simulink model "sudoku_PP_CEX2"  (R2017b)
settings: Solver=FixedStepDiscrete  StartTime=0.0  StopTime=10.0  FixedStep=0.200000  RelTol=1e-3
model workspace (MAT data in the model file):
  MCOS : class17 (value not decoded)
  already_pp = 1
  compositionalMap : struct (value not decoded)
  MCOS : class17 (value not decoded)
  MCOS : class17 (value not decoded)
  verificationResults : struct (value not decoded)
undefined symbols (not defined in the file): contractAfterSimulation, ContractAssumeBlock, contractBeforeSimulation, ContractBlock, ContractGuaranteeBlock, ContractValidatorBlock, saveValidatorParameters
(part 7 of 17)

== system sudoku_PP_CEX2/contract/guarantee/RowsValid/ForEach_newline_Subsystem/ForEach3/Vectorisvalid ==
  In1 : Inport
  Compare To Constant : Subsystem  AncestorBlock=|  TreatAsAtomicUnit=on  mask(Compare To Constant){relop===, const=1, OutDataTypeStr=boolean, ZeroCross=on}
      | simulink/Logic and Bit
      | Operations/Compare
      | To Constant
      mask prompts: relop "Simulink:masks:Operator_MP"; const "Simulink:masks:ConstantValue_MP"; OutDataTypeStr "Simulink:masks:OutputDataType_MP"; ZeroCross "Simulink:masks:EnableZerocrossingDetection_MP"
      mask help: Simulink:masks:CompareToConstant_MD
      mask init: same as sudoku_PP_CEX2/contract/guarantee/ColsValid/ForEach_newline_Subsystem/ForEach1/Vectorisvalid/Compare To Constant
      mask TypeOptions relop: == | ~= | < | <= | >= | >
      mask TypeOptions OutDataTypeStr: Simulink:masks:uint8 | Simulink:masks:boolean
      mask Callback ZeroCross: sl('zeroCrossEnable', gcbh);
      mask Display: disp(str)
  Compare To Constant1 : Subsystem  AncestorBlock=|  TreatAsAtomicUnit=on  mask(Compare To Constant){relop===, const=1, OutDataTypeStr=boolean, ZeroCross=on}
      | simulink/Logic and Bit
      | Operations/Compare
      | To Constant
      mask prompts: relop "Simulink:masks:Operator_MP"; const "Simulink:masks:ConstantValue_MP"; OutDataTypeStr "Simulink:masks:OutputDataType_MP"; ZeroCross "Simulink:masks:EnableZerocrossingDetection_MP"
      mask help: Simulink:masks:CompareToConstant_MD
      mask init: same as sudoku_PP_CEX2/contract/guarantee/ColsValid/ForEach_newline_Subsystem/ForEach1/Vectorisvalid/Compare To Constant
      mask TypeOptions relop: == | ~= | < | <= | >= | >
      mask TypeOptions OutDataTypeStr: Simulink:masks:uint8 | Simulink:masks:boolean
      mask Callback ZeroCross: sl('zeroCrossEnable', gcbh);
      mask Display: disp(str)
  Compare To Constant2 : Subsystem  AncestorBlock=|  TreatAsAtomicUnit=on  mask(Compare To Constant){relop===, const=1, OutDataTypeStr=boolean, ZeroCross=on}
      | simulink/Logic and Bit
      | Operations/Compare
      | To Constant
      mask prompts: relop "Simulink:masks:Operator_MP"; const "Simulink:masks:ConstantValue_MP"; OutDataTypeStr "Simulink:masks:OutputDataType_MP"; ZeroCross "Simulink:masks:EnableZerocrossingDetection_MP"
      mask help: Simulink:masks:CompareToConstant_MD
      mask init: same as sudoku_PP_CEX2/contract/guarantee/ColsValid/ForEach_newline_Subsystem/ForEach1/Vectorisvalid/Compare To Constant
      mask TypeOptions relop: == | ~= | < | <= | >= | >
      mask TypeOptions OutDataTypeStr: Simulink:masks:uint8 | Simulink:masks:boolean
      mask Callback ZeroCross: sl('zeroCrossEnable', gcbh);
      mask Display: disp(str)
  Compare To Constant3 : Subsystem  AncestorBlock=|  TreatAsAtomicUnit=on  mask(Compare To Constant){relop===, const=1, OutDataTypeStr=boolean, ZeroCross=on}
      | simulink/Logic and Bit
      | Operations/Compare
      | To Constant
      mask prompts: relop "Simulink:masks:Operator_MP"; const "Simulink:masks:ConstantValue_MP"; OutDataTypeStr "Simulink:masks:OutputDataType_MP"; ZeroCross "Simulink:masks:EnableZerocrossingDetection_MP"
      mask help: Simulink:masks:CompareToConstant_MD
      mask init: same as sudoku_PP_CEX2/contract/guarantee/ColsValid/ForEach_newline_Subsystem/ForEach1/Vectorisvalid/Compare To Constant
      mask TypeOptions relop: == | ~= | < | <= | >= | >
      mask TypeOptions OutDataTypeStr: Simulink:masks:uint8 | Simulink:masks:boolean
      mask Callback ZeroCross: sl('zeroCrossEnable', gcbh);
      mask Display: disp(str)
  Compare To Constant4 : Subsystem  AncestorBlock=|  TreatAsAtomicUnit=on  mask(Compare To Constant){relop===, const=1, OutDataTypeStr=boolean, ZeroCross=on}
      | simulink/Logic and Bit
      | Operations/Compare
      | To Constant
      mask prompts: relop "Simulink:masks:Operator_MP"; const "Simulink:masks:ConstantValue_MP"; OutDataTypeStr "Simulink:masks:OutputDataType_MP"; ZeroCross "Simulink:masks:EnableZerocrossingDetection_MP"
      mask help: Simulink:masks:CompareToConstant_MD
      mask init: same as sudoku_PP_CEX2/contract/guarantee/ColsValid/ForEach_newline_Subsystem/ForEach1/Vectorisvalid/Compare To Constant
      mask TypeOptions relop: == | ~= | < | <= | >= | >
      mask TypeOptions OutDataTypeStr: Simulink:masks:uint8 | Simulink:masks:boolean
      mask Callback ZeroCross: sl('zeroCrossEnable', gcbh);
      mask Display: disp(str)
  Compare To Constant5 : Subsystem  AncestorBlock=|  TreatAsAtomicUnit=on  mask(Compare To Constant){relop===, const=1, OutDataTypeStr=boolean, ZeroCross=on}
      | simulink/Logic and Bit
      | Operations/Compare
      | To Constant
      mask prompts: relop "Simulink:masks:Operator_MP"; const "Simulink:masks:ConstantValue_MP"; OutDataTypeStr "Simulink:masks:OutputDataType_MP"; ZeroCross "Simulink:masks:EnableZerocrossingDetection_MP"
      mask help: Simulink:masks:CompareToConstant_MD
      mask init: same as sudoku_PP_CEX2/contract/guarantee/ColsValid/ForEach_newline_Subsystem/ForEach1/Vectorisvalid/Compare To Constant
      mask TypeOptions relop: == | ~= | < | <= | >= | >
      mask TypeOptions OutDataTypeStr: Simulink:masks:uint8 | Simulink:masks:boolean
      mask Callback ZeroCross: sl('zeroCrossEnable', gcbh);
      mask Display: disp(str)
  Compare To Constant6 : Subsystem  AncestorBlock=|  TreatAsAtomicUnit=on  mask(Compare To Constant){relop===, const=1, OutDataTypeStr=boolean, ZeroCross=on}
      | simulink/Logic and Bit
      | Operations/Compare
      | To Constant
      mask prompts: relop "Simulink:masks:Operator_MP"; const "Simulink:masks:ConstantValue_MP"; OutDataTypeStr "Simulink:masks:OutputDataType_MP"; ZeroCross "Simulink:masks:EnableZerocrossingDetection_MP"
      mask help: Simulink:masks:CompareToConstant_MD
      mask init: same as sudoku_PP_CEX2/contract/guarantee/ColsValid/ForEach_newline_Subsystem/ForEach1/Vectorisvalid/Compare To Constant
      mask TypeOptions relop: == | ~= | < | <= | >= | >
      mask TypeOptions OutDataTypeStr: Simulink:masks:uint8 | Simulink:masks:boolean
      mask Callback ZeroCross: sl('zeroCrossEnable', gcbh);
      mask Display: disp(str)
  Compare To Constant7 : Subsystem  AncestorBlock=|  TreatAsAtomicUnit=on  mask(Compare To Constant){relop===, const=1, OutDataTypeStr=boolean, ZeroCross=on}
      | simulink/Logic and Bit
      | Operations/Compare
      | To Constant
      mask prompts: relop "Simulink:masks:Operator_MP"; const "Simulink:masks:ConstantValue_MP"; OutDataTypeStr "Simulink:masks:OutputDataType_MP"; ZeroCross "Simulink:masks:EnableZerocrossingDetection_MP"
      mask help: Simulink:masks:CompareToConstant_MD
      mask init: same as sudoku_PP_CEX2/contract/guarantee/ColsValid/ForEach_newline_Subsystem/ForEach1/Vectorisvalid/Compare To Constant
      mask TypeOptions relop: == | ~= | < | <= | >= | >
      mask TypeOptions OutDataTypeStr: Simulink:masks:uint8 | Simulink:masks:boolean
      mask Callback ZeroCross: sl('zeroCrossEnable', gcbh);
      mask Display: disp(str)
  Compare To Constant8 : Subsystem  AncestorBlock=|  TreatAsAtomicUnit=on  mask(Compare To Constant){relop=>=, const=1, OutDataTypeStr=boolean, ZeroCross=on}
      | simulink/Logic and Bit
      | Operations/Compare
      | To Constant
      mask prompts: relop "Simulink:masks:Operator_MP"; const "Simulink:masks:ConstantValue_MP"; OutDataTypeStr "Simulink:masks:OutputDataType_MP"; ZeroCross "Simulink:masks:EnableZerocrossingDetection_MP"
      mask help: Simulink:masks:CompareToConstant_MD
      mask init: same as sudoku_PP_CEX2/contract/guarantee/ColsValid/ForEach_newline_Subsystem/ForEach1/Vectorisvalid/Compare To Constant
      mask TypeOptions relop: == | ~= | < | <= | >= | >
      mask TypeOptions OutDataTypeStr: Simulink:masks:uint8 | Simulink:masks:boolean
      mask Callback ZeroCross: sl('zeroCrossEnable', gcbh);
      mask Display: disp(str)
  Compare To Constant9 : Subsystem  AncestorBlock=|  TreatAsAtomicUnit=on  mask(Compare To Constant){relop=<=, const=9, OutDataTypeStr=boolean, ZeroCross=on}
      | simulink/Logic and Bit
      | Operations/Compare
      | To Constant
      mask prompts: relop "Simulink:masks:Operator_MP"; const "Simulink:masks:ConstantValue_MP"; OutDataTypeStr "Simulink:masks:OutputDataType_MP"; ZeroCross "Simulink:masks:EnableZerocrossingDetection_MP"
      mask help: Simulink:masks:CompareToConstant_MD
      mask init: same as sudoku_PP_CEX2/contract/guarantee/ColsValid/ForEach_newline_Subsystem/ForEach1/Vectorisvalid/Compare To Constant
      mask TypeOptions relop: == | ~= | < | <= | >= | >
      mask TypeOptions OutDataTypeStr: Simulink:masks:uint8 | Simulink:masks:boolean
      mask Callback ZeroCross: sl('zeroCrossEnable', gcbh);
      mask Display: disp(str)
  DataTypeConversion : DataTypeConversion  OutDataTypeStr=double
  Fcn : Fcn  Expr=u(1) != u(2) && u(1) != u(3) && u(1) != u(4) && u(1) != u(5) && u(1) != u(6) && u(1) != u(7) && u(1) != u(8) && u(1) != u(9)
  Fcn1 : Fcn  Expr=u(2) != u(3) && u(2) != u(4) && u(2) != u(5) && u(2) != u(6) && u(2) != u(7) && u(2) != u(8) && u(2) != u(9)
  Fcn2 : Fcn  Expr=u(3) != u(4) && u(3) != u(5) && u(3) != u(6) && u(3) != u(7) && u(3) != u(8) && u(3) != u(9)
  Fcn3 : Fcn  Expr=u(4) != u(5) && u(4) != u(6) && u(4) != u(7) && u(4) != u(8) && u(4) != u(9)
  Fcn4 : Fcn  Expr=u(5) != u(6) && u(5) != u(7) && u(5) != u(8) && u(5) != u(9)
  Fcn5 : Fcn  Expr=u(6) != u(7) && u(6) != u(8) && u(6) != u(9)
  Fcn6 : Fcn  Expr=u(7) != u(8) && u(7) != u(9)
  Fcn7 : Fcn  Expr=u(8) != u(9)
  Logical_newline_Operator : Logic  Inputs=10  AllPortsSameDT=off  OutDataTypeStr=boolean
  Logical_newline_Operator1 : Logic  Inputs=1  AllPortsSameDT=off  OutDataTypeStr=boolean
  Logical_newline_Operator2 : Logic  Inputs=1  AllPortsSameDT=off  OutDataTypeStr=boolean
  Out1 : Outport
  wires:
  Logical_newline_Operator/1 -> Out1/1
  Compare To Constant9/1(y) -> Logical_newline_Operator2/1
  Compare To Constant8/1(y) -> Logical_newline_Operator1/1
  Logical_newline_Operator2/1 -> Logical_newline_Operator/10
  Logical_newline_Operator1/1 -> Logical_newline_Operator/9
  Compare To Constant7/1(y) -> Logical_newline_Operator/8
  Compare To Constant6/1(y) -> Logical_newline_Operator/7
  Compare To Constant5/1(y) -> Logical_newline_Operator/6
  Compare To Constant4/1(y) -> Logical_newline_Operator/5
  Compare To Constant3/1(y) -> Logical_newline_Operator/4
  Compare To Constant2/1(y) -> Logical_newline_Operator/3
  Compare To Constant1/1(y) -> Logical_newline_Operator/2
  Compare To Constant/1(y) -> Logical_newline_Operator/1
  In1/1 -> DataTypeConversion/1
  Fcn7/1 -> Compare To Constant7/1(u)
  Fcn6/1 -> Compare To Constant6/1(u)
  Fcn5/1 -> Compare To Constant5/1(u)
  Fcn4/1 -> Compare To Constant4/1(u)
  Fcn3/1 -> Compare To Constant3/1(u)
  Fcn2/1 -> Compare To Constant2/1(u)
  Fcn1/1 -> Compare To Constant1/1(u)
  Fcn/1 -> Compare To Constant/1(u)
  DataTypeConversion/1 -> Fcn7/1, Fcn6/1, Fcn5/1, Fcn4/1, Fcn3/1, Fcn2/1, Fcn1/1, Fcn/1, Compare To Constant9/1(u), Compare To Constant8/1(u)

== system sudoku_PP_CEX2/contract/guarantee/RowsValid/ForEach_newline_Subsystem/ForEach4/Vectorisvalid ==
  In1 : Inport
  Compare To Constant : Subsystem  AncestorBlock=|  TreatAsAtomicUnit=on  mask(Compare To Constant){relop===, const=1, OutDataTypeStr=boolean, ZeroCross=on}
      | simulink/Logic and Bit
      | Operations/Compare
      | To Constant
      mask prompts: relop "Simulink:masks:Operator_MP"; const "Simulink:masks:ConstantValue_MP"; OutDataTypeStr "Simulink:masks:OutputDataType_MP"; ZeroCross "Simulink:masks:EnableZerocrossingDetection_MP"
      mask help: Simulink:masks:CompareToConstant_MD
      mask init: same as sudoku_PP_CEX2/contract/guarantee/ColsValid/ForEach_newline_Subsystem/ForEach1/Vectorisvalid/Compare To Constant
      mask TypeOptions relop: == | ~= | < | <= | >= | >
      mask TypeOptions OutDataTypeStr: Simulink:masks:uint8 | Simulink:masks:boolean
      mask Callback ZeroCross: sl('zeroCrossEnable', gcbh);
      mask Display: disp(str)
  Compare To Constant1 : Subsystem  AncestorBlock=|  TreatAsAtomicUnit=on  mask(Compare To Constant){relop===, const=1, OutDataTypeStr=boolean, ZeroCross=on}
      | simulink/Logic and Bit
      | Operations/Compare
      | To Constant
      mask prompts: relop "Simulink:masks:Operator_MP"; const "Simulink:masks:ConstantValue_MP"; OutDataTypeStr "Simulink:masks:OutputDataType_MP"; ZeroCross "Simulink:masks:EnableZerocrossingDetection_MP"
      mask help: Simulink:masks:CompareToConstant_MD
      mask init: same as sudoku_PP_CEX2/contract/guarantee/ColsValid/ForEach_newline_Subsystem/ForEach1/Vectorisvalid/Compare To Constant
      mask TypeOptions relop: == | ~= | < | <= | >= | >
      mask TypeOptions OutDataTypeStr: Simulink:masks:uint8 | Simulink:masks:boolean
      mask Callback ZeroCross: sl('zeroCrossEnable', gcbh);
      mask Display: disp(str)
  Compare To Constant2 : Subsystem  AncestorBlock=|  TreatAsAtomicUnit=on  mask(Compare To Constant){relop===, const=1, OutDataTypeStr=boolean, ZeroCross=on}
      | simulink/Logic and Bit
      | Operations/Compare
      | To Constant
      mask prompts: relop "Simulink:masks:Operator_MP"; const "Simulink:masks:ConstantValue_MP"; OutDataTypeStr "Simulink:masks:OutputDataType_MP"; ZeroCross "Simulink:masks:EnableZerocrossingDetection_MP"
      mask help: Simulink:masks:CompareToConstant_MD
      mask init: same as sudoku_PP_CEX2/contract/guarantee/ColsValid/ForEach_newline_Subsystem/ForEach1/Vectorisvalid/Compare To Constant
      mask TypeOptions relop: == | ~= | < | <= | >= | >
      mask TypeOptions OutDataTypeStr: Simulink:masks:uint8 | Simulink:masks:boolean
      mask Callback ZeroCross: sl('zeroCrossEnable', gcbh);
      mask Display: disp(str)
  Compare To Constant3 : Subsystem  AncestorBlock=|  TreatAsAtomicUnit=on  mask(Compare To Constant){relop===, const=1, OutDataTypeStr=boolean, ZeroCross=on}
      | simulink/Logic and Bit
      | Operations/Compare
      | To Constant
      mask prompts: relop "Simulink:masks:Operator_MP"; const "Simulink:masks:ConstantValue_MP"; OutDataTypeStr "Simulink:masks:OutputDataType_MP"; ZeroCross "Simulink:masks:EnableZerocrossingDetection_MP"
      mask help: Simulink:masks:CompareToConstant_MD
      mask init: same as sudoku_PP_CEX2/contract/guarantee/ColsValid/ForEach_newline_Subsystem/ForEach1/Vectorisvalid/Compare To Constant
      mask TypeOptions relop: == | ~= | < | <= | >= | >
      mask TypeOptions OutDataTypeStr: Simulink:masks:uint8 | Simulink:masks:boolean
      mask Callback ZeroCross: sl('zeroCrossEnable', gcbh);
      mask Display: disp(str)
  Compare To Constant4 : Subsystem  AncestorBlock=|  TreatAsAtomicUnit=on  mask(Compare To Constant){relop===, const=1, OutDataTypeStr=boolean, ZeroCross=on}
      | simulink/Logic and Bit
      | Operations/Compare
      | To Constant
      mask prompts: relop "Simulink:masks:Operator_MP"; const "Simulink:masks:ConstantValue_MP"; OutDataTypeStr "Simulink:masks:OutputDataType_MP"; ZeroCross "Simulink:masks:EnableZerocrossingDetection_MP"
      mask help: Simulink:masks:CompareToConstant_MD
      mask init: same as sudoku_PP_CEX2/contract/guarantee/ColsValid/ForEach_newline_Subsystem/ForEach1/Vectorisvalid/Compare To Constant
      mask TypeOptions relop: == | ~= | < | <= | >= | >
      mask TypeOptions OutDataTypeStr: Simulink:masks:uint8 | Simulink:masks:boolean
      mask Callback ZeroCross: sl('zeroCrossEnable', gcbh);
      mask Display: disp(str)
  Compare To Constant5 : Subsystem  AncestorBlock=|  TreatAsAtomicUnit=on  mask(Compare To Constant){relop===, const=1, OutDataTypeStr=boolean, ZeroCross=on}
      | simulink/Logic and Bit
      | Operations/Compare
      | To Constant
      mask prompts: relop "Simulink:masks:Operator_MP"; const "Simulink:masks:ConstantValue_MP"; OutDataTypeStr "Simulink:masks:OutputDataType_MP"; ZeroCross "Simulink:masks:EnableZerocrossingDetection_MP"
      mask help: Simulink:masks:CompareToConstant_MD
      mask init: same as sudoku_PP_CEX2/contract/guarantee/ColsValid/ForEach_newline_Subsystem/ForEach1/Vectorisvalid/Compare To Constant
      mask TypeOptions relop: == | ~= | < | <= | >= | >
      mask TypeOptions OutDataTypeStr: Simulink:masks:uint8 | Simulink:masks:boolean
      mask Callback ZeroCross: sl('zeroCrossEnable', gcbh);
      mask Display: disp(str)
  Compare To Constant6 : Subsystem  AncestorBlock=|  TreatAsAtomicUnit=on  mask(Compare To Constant){relop===, const=1, OutDataTypeStr=boolean, ZeroCross=on}
      | simulink/Logic and Bit
      | Operations/Compare
      | To Constant
      mask prompts: relop "Simulink:masks:Operator_MP"; const "Simulink:masks:ConstantValue_MP"; OutDataTypeStr "Simulink:masks:OutputDataType_MP"; ZeroCross "Simulink:masks:EnableZerocrossingDetection_MP"
      mask help: Simulink:masks:CompareToConstant_MD
      mask init: same as sudoku_PP_CEX2/contract/guarantee/ColsValid/ForEach_newline_Subsystem/ForEach1/Vectorisvalid/Compare To Constant
      mask TypeOptions relop: == | ~= | < | <= | >= | >
      mask TypeOptions OutDataTypeStr: Simulink:masks:uint8 | Simulink:masks:boolean
      mask Callback ZeroCross: sl('zeroCrossEnable', gcbh);
      mask Display: disp(str)
  Compare To Constant7 : Subsystem  AncestorBlock=|  TreatAsAtomicUnit=on  mask(Compare To Constant){relop===, const=1, OutDataTypeStr=boolean, ZeroCross=on}
      | simulink/Logic and Bit
      | Operations/Compare
      | To Constant
      mask prompts: relop "Simulink:masks:Operator_MP"; const "Simulink:masks:ConstantValue_MP"; OutDataTypeStr "Simulink:masks:OutputDataType_MP"; ZeroCross "Simulink:masks:EnableZerocrossingDetection_MP"
      mask help: Simulink:masks:CompareToConstant_MD
      mask init: same as sudoku_PP_CEX2/contract/guarantee/ColsValid/ForEach_newline_Subsystem/ForEach1/Vectorisvalid/Compare To Constant
      mask TypeOptions relop: == | ~= | < | <= | >= | >
      mask TypeOptions OutDataTypeStr: Simulink:masks:uint8 | Simulink:masks:boolean
      mask Callback ZeroCross: sl('zeroCrossEnable', gcbh);
      mask Display: disp(str)
  Compare To Constant8 : Subsystem  AncestorBlock=|  TreatAsAtomicUnit=on  mask(Compare To Constant){relop=>=, const=1, OutDataTypeStr=boolean, ZeroCross=on}
      | simulink/Logic and Bit
      | Operations/Compare
      | To Constant
      mask prompts: relop "Simulink:masks:Operator_MP"; const "Simulink:masks:ConstantValue_MP"; OutDataTypeStr "Simulink:masks:OutputDataType_MP"; ZeroCross "Simulink:masks:EnableZerocrossingDetection_MP"
      mask help: Simulink:masks:CompareToConstant_MD
      mask init: same as sudoku_PP_CEX2/contract/guarantee/ColsValid/ForEach_newline_Subsystem/ForEach1/Vectorisvalid/Compare To Constant
      mask TypeOptions relop: == | ~= | < | <= | >= | >
      mask TypeOptions OutDataTypeStr: Simulink:masks:uint8 | Simulink:masks:boolean
      mask Callback ZeroCross: sl('zeroCrossEnable', gcbh);
      mask Display: disp(str)
  Compare To Constant9 : Subsystem  AncestorBlock=|  TreatAsAtomicUnit=on  mask(Compare To Constant){relop=<=, const=9, OutDataTypeStr=boolean, ZeroCross=on}
      | simulink/Logic and Bit
      | Operations/Compare
      | To Constant
      mask prompts: relop "Simulink:masks:Operator_MP"; const "Simulink:masks:ConstantValue_MP"; OutDataTypeStr "Simulink:masks:OutputDataType_MP"; ZeroCross "Simulink:masks:EnableZerocrossingDetection_MP"
      mask help: Simulink:masks:CompareToConstant_MD
      mask init: same as sudoku_PP_CEX2/contract/guarantee/ColsValid/ForEach_newline_Subsystem/ForEach1/Vectorisvalid/Compare To Constant
      mask TypeOptions relop: == | ~= | < | <= | >= | >
      mask TypeOptions OutDataTypeStr: Simulink:masks:uint8 | Simulink:masks:boolean
      mask Callback ZeroCross: sl('zeroCrossEnable', gcbh);
      mask Display: disp(str)
  DataTypeConversion : DataTypeConversion  OutDataTypeStr=double
  Fcn : Fcn  Expr=u(1) != u(2) && u(1) != u(3) && u(1) != u(4) && u(1) != u(5) && u(1) != u(6) && u(1) != u(7) && u(1) != u(8) && u(1) != u(9)
  Fcn1 : Fcn  Expr=u(2) != u(3) && u(2) != u(4) && u(2) != u(5) && u(2) != u(6) && u(2) != u(7) && u(2) != u(8) && u(2) != u(9)
  Fcn2 : Fcn  Expr=u(3) != u(4) && u(3) != u(5) && u(3) != u(6) && u(3) != u(7) && u(3) != u(8) && u(3) != u(9)
  Fcn3 : Fcn  Expr=u(4) != u(5) && u(4) != u(6) && u(4) != u(7) && u(4) != u(8) && u(4) != u(9)
  Fcn4 : Fcn  Expr=u(5) != u(6) && u(5) != u(7) && u(5) != u(8) && u(5) != u(9)
  Fcn5 : Fcn  Expr=u(6) != u(7) && u(6) != u(8) && u(6) != u(9)
  Fcn6 : Fcn  Expr=u(7) != u(8) && u(7) != u(9)
  Fcn7 : Fcn  Expr=u(8) != u(9)
  Logical_newline_Operator : Logic  Inputs=10  AllPortsSameDT=off  OutDataTypeStr=boolean
  Logical_newline_Operator1 : Logic  Inputs=1  AllPortsSameDT=off  OutDataTypeStr=boolean
  Logical_newline_Operator2 : Logic  Inputs=1  AllPortsSameDT=off  OutDataTypeStr=boolean
  Out1 : Outport
  wires:
  Logical_newline_Operator/1 -> Out1/1
  Compare To Constant9/1(y) -> Logical_newline_Operator2/1
  Compare To Constant8/1(y) -> Logical_newline_Operator1/1
  Logical_newline_Operator2/1 -> Logical_newline_Operator/10
  Logical_newline_Operator1/1 -> Logical_newline_Operator/9
  Compare To Constant7/1(y) -> Logical_newline_Operator/8
  Compare To Constant6/1(y) -> Logical_newline_Operator/7
  Compare To Constant5/1(y) -> Logical_newline_Operator/6
  Compare To Constant4/1(y) -> Logical_newline_Operator/5
  Compare To Constant3/1(y) -> Logical_newline_Operator/4
  Compare To Constant2/1(y) -> Logical_newline_Operator/3
  Compare To Constant1/1(y) -> Logical_newline_Operator/2
  Compare To Constant/1(y) -> Logical_newline_Operator/1
  In1/1 -> DataTypeConversion/1
  Fcn7/1 -> Compare To Constant7/1(u)
  Fcn6/1 -> Compare To Constant6/1(u)
  Fcn5/1 -> Compare To Constant5/1(u)
  Fcn4/1 -> Compare To Constant4/1(u)
  Fcn3/1 -> Compare To Constant3/1(u)
  Fcn2/1 -> Compare To Constant2/1(u)
  Fcn1/1 -> Compare To Constant1/1(u)
  Fcn/1 -> Compare To Constant/1(u)
  DataTypeConversion/1 -> Fcn7/1, Fcn6/1, Fcn5/1, Fcn4/1, Fcn3/1, Fcn2/1, Fcn1/1, Fcn/1, Compare To Constant9/1(u), Compare To Constant8/1(u)
